simulink model "asw_28_simulator"  (R2018b)
settings: Solver=ode4  StartTime=0.0  StopTime=100  FixedStep=0.001  RelTol=1e-3
undefined symbols (not defined in the file): Earth, WGS84
libraries: simulink x4, aerolibutil x3, sharedtransform x2, aerolibtransform2 x2, aerolibfltsims x1, sharedutil x1
settings Model: Creator=benma  LastModifiedBy=benma

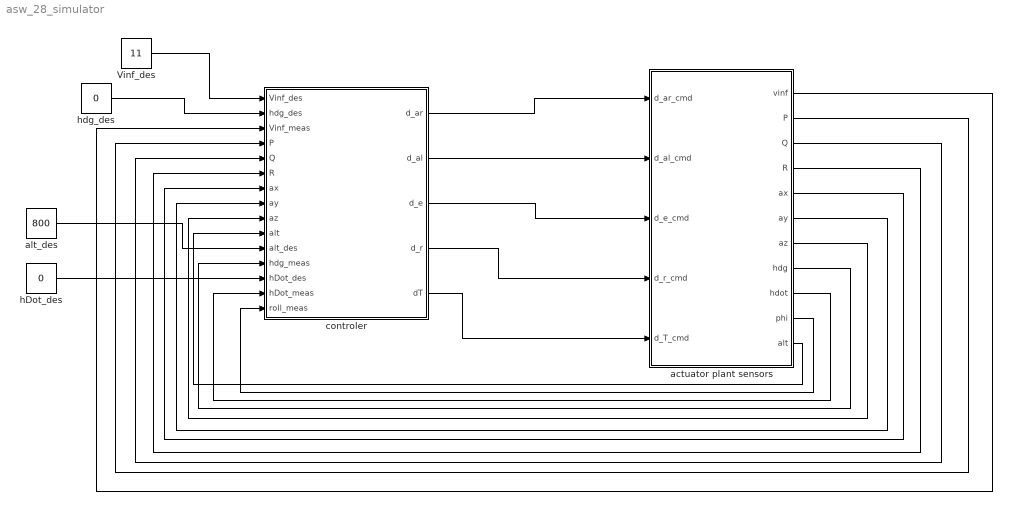
== system asw_28_simulator ==
  Vinf_des : Constant  Value=11
  actuator plant sensors : Subsystem
  alt_des : Constant  Value=800
  controler : Subsystem
  hDot_des : Constant  Value=0
  hdg_des : Constant  Value=0
  wires:
  controler/1(d_ar) -> actuator plant sensors/1(d_ar_cmd)
  controler/3(d_e) -> actuator plant sensors/3(d_e_cmd)
  controler/2(d_al) -> actuator plant sensors/2(d_al_cmd)
  controler/4(d_r) -> actuator plant sensors/4(d_r_cmd)
  hDot_des/1 -> controler/13(hDot_des)
  actuator plant sensors/9(hdot) -> controler/14(hDot_meas)
  actuator plant sensors/5(ax) -> controler/7(ax)
  actuator plant sensors/10(phi) -> controler/15(roll_meas)
  actuator plant sensors/3(Q) -> controler/5(Q)
  actuator plant sensors/4(R) -> controler/6(R)
  actuator plant sensors/2(P) -> controler/4(P)
  actuator plant sensors/6(ay) -> controler/8(ay)
  actuator plant sensors/1(vinf) -> controler/3(Vinf_meas)
  actuator plant sensors/7(az) -> controler/9(az)
  actuator plant sensors/8(hdg) -> controler/12(hdg_meas)
  hdg_des/1 -> controler/2(hdg_des)
  Vinf_des/1 -> controler/1(Vinf_des)
  actuator plant sensors/11(alt) -> controler/10(alt)
  alt_des/1 -> controler/11(alt_des)
  controler/5(dT) -> actuator plant sensors/5(d_T_cmd)

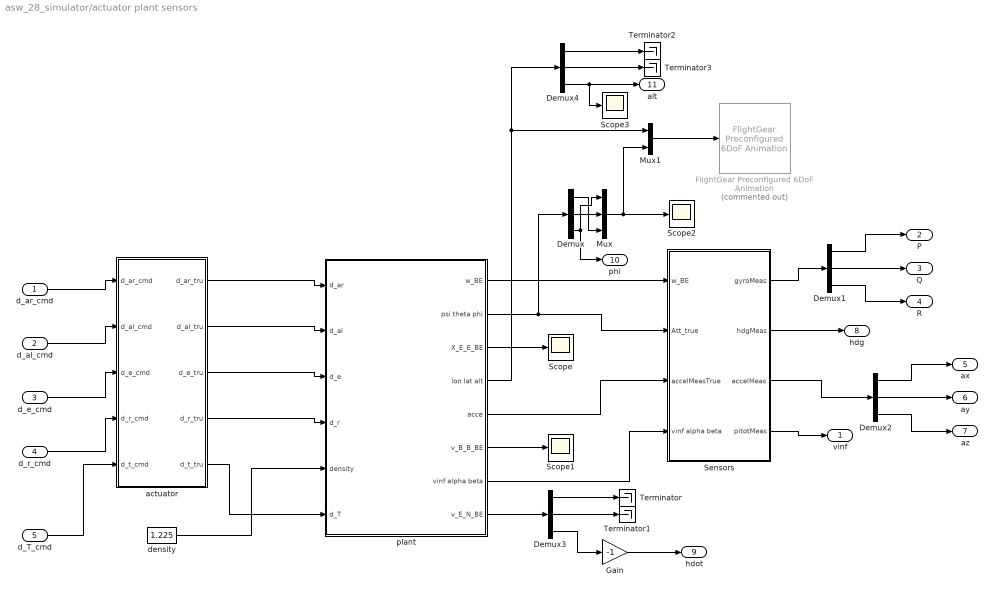
== system asw_28_simulator/actuator plant sensors ==
  d_ar_cmd : Inport
  d_al_cmd : Inport  Port=2
  d_e_cmd : Inport  Port=3
  d_r_cmd : Inport  Port=4
  d_T_cmd : Inport  Port=5
  Demux{,1..4} (5 alike) : Demux  Outputs=3
  FlightGear Preconfigured 6DoF Animation : aerolibfltsims/FlightGear Preconfigured 6DoF Animation  Commented=on  xFlightGearVersion=v2018.1  DestinationIpAddress=127.0.0.1  DestinationPort=5502  SampleTime=1/30  packetVersion=24
      settings: SourceProductName=Aerospace Blockset
  Gain : Gain  Gain=-1
  Mux : Mux  Inputs=3
  Mux1 : Mux  Inputs=2
  Scope{,1..3} (4 alike) : Scope
  Sensors : Subsystem
  Terminator{,1..3} (4 alike) : Terminator
  actuator : Subsystem
  density : Constant  Value=1.225
  plant : Subsystem
  vinf : Outport
  P : Outport  Port=2
  Q : Outport  Port=3
  R : Outport  Port=4
  ax : Outport  Port=5
  ay : Outport  Port=6
  az : Outport  Port=7
  hdg : Outport  Port=8
  hdot : Outport  Port=9
  phi : Outport  Port=10
  alt : Outport  Port=11
  wires:
  plant/6(v_B_B_BE) -> Scope1/1
  Demux/1 -> Mux/3
  Demux2/1 -> ax/1
  plant/4(lon lat alt) -> Mux1/1, Demux4/1
  plant/5(acce) -> Sensors/3(accelMeasTrue)
  d_e_cmd/1 -> actuator/3(d_e_cmd)
  Sensors/3(accelMeas) -> Demux2/1
  d_ar_cmd/1 -> actuator/1(d_ar_cmd)
  Sensors/2(hdgMeas) -> hdg/1
  Mux1/1 -> FlightGear Preconfigured 6DoF Animation/1
  actuator/3(d_e_tru) -> plant/3(d_e)
  plant/7(vinf alpha beta) -> Sensors/4(vinf alpha beta)
  Demux1/1 -> P/1
  d_r_cmd/1 -> actuator/4(d_r_cmd)
  actuator/1(d_ar_tru) -> plant/1(d_ar)
  plant/3(X_E_E_BE) -> Scope/1
  Demux1/3 -> R/1
  plant/1(w_BE) -> Sensors/1(w_BE)
  density/1 -> plant/5(density)
  Sensors/1(gyroMeas) -> Demux1/1
  Mux/1 -> Scope2/1, Mux1/2
  actuator/2(d_al_tru) -> plant/2(d_al)
  Demux/2 -> Mux/2
  Demux2/2 -> ay/1
  Demux1/2 -> Q/1
  plant/2(psi theta phi) -> Sensors/2(Att_true), Demux/1
  Sensors/4(pitotMeas) -> vinf/1
  Demux2/3 -> az/1
  d_al_cmd/1 -> actuator/2(d_al_cmd)
  actuator/4(d_r_tru) -> plant/4(d_r)
  Demux/3 -> phi/1, Mux/1
  plant/8(v_E_N_BE) -> Demux3/1
  Demux3/1 -> Terminator/1
  Demux3/2 -> Terminator1/1
  Demux3/3 -> Gain/1
  Gain/1 -> hdot/1
  Demux4/1 -> Terminator2/1
  Demux4/2 -> Terminator3/1
  Demux4/3 -> Scope3/1, alt/1
  d_T_cmd/1 -> actuator/5(d_t_cmd)
  actuator/5(d_t_tru) -> plant/6(d_T)

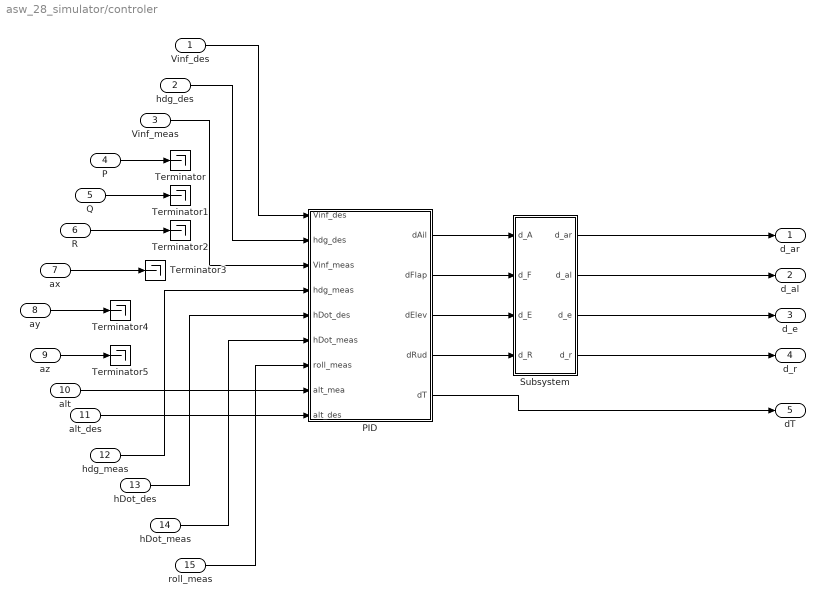
== system asw_28_simulator/controler ==
  Vinf_des : Inport
  hdg_des : Inport  Port=2
  Vinf_meas : Inport  Port=3
  P : Inport  Port=4
  Q : Inport  Port=5
  R : Inport  Port=6
  ax : Inport  Port=7
  ay : Inport  Port=8
  az : Inport  Port=9
  alt : Inport  Port=10
  alt_des : Inport  Port=11
  hdg_meas : Inport  Port=12
  hDot_des : Inport  Port=13
  hDot_meas : Inport  Port=14
  roll_meas : Inport  Port=15
  PID : Subsystem
  Subsystem : Subsystem
  Terminator{,1..5} (6 alike) : Terminator
  d_ar : Outport
  d_al : Outport  Port=2
  d_e : Outport  Port=3
  d_r : Outport  Port=4
  dT : Outport  Port=5
  wires:
  hdg_des/1 -> PID/2(hdg_des)
  Subsystem/2(d_al) -> d_al/1
  Vinf_des/1 -> PID/1(Vinf_des)
  Subsystem/3(d_e) -> d_e/1
  Vinf_meas/1 -> PID/3(Vinf_meas)
  hDot_des/1 -> PID/5(hDot_des)
  roll_meas/1 -> PID/7(roll_meas)
  Subsystem/4(d_r) -> d_r/1
  hdg_meas/1 -> PID/4(hdg_meas)
  PID/2(dFlap) -> Subsystem/2(d_F)
  Subsystem/1(d_ar) -> d_ar/1
  PID/4(dRud) -> Subsystem/4(d_R)
  PID/5(dT) -> dT/1
  PID/1(dAil) -> Subsystem/1(d_A)
  hDot_meas/1 -> PID/6(hDot_meas)
  PID/3(dElev) -> Subsystem/3(d_E)
  P/1 -> Terminator/1
  Q/1 -> Terminator1/1
  R/1 -> Terminator2/1
  ax/1 -> Terminator3/1
  ay/1 -> Terminator4/1
  az/1 -> Terminator5/1
  alt/1 -> PID/8(alt_mea)
  alt_des/1 -> PID/9(alt_des)

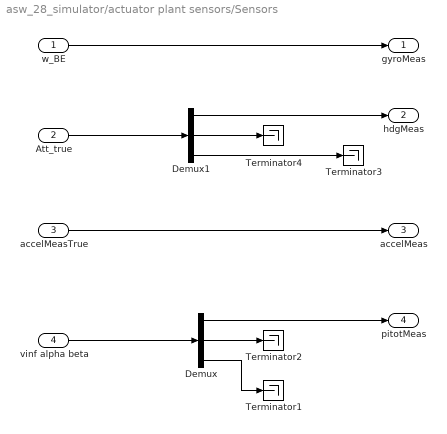
== system asw_28_simulator/actuator plant sensors/Sensors ==
  w_BE : Inport
  Att_true : Inport  Port=2
  accelMeasTrue : Inport  Port=3
  vinf alpha beta : Inport  Port=4
  Demux : Demux  Outputs=3
  Demux1 : Demux  Outputs=3
  Terminator{1..4} (4 alike) : Terminator
  gyroMeas : Outport
  hdgMeas : Outport  Port=2
  accelMeas : Outport  Port=3
  pitotMeas : Outport  Port=4
  wires:
  w_BE/1 -> gyroMeas/1
  vinf alpha beta/1 -> Demux/1
  Demux/3 -> Terminator1/1
  Demux/2 -> Terminator2/1
  Demux/1 -> pitotMeas/1
  accelMeasTrue/1 -> accelMeas/1
  Att_true/1 -> Demux1/1
  Demux1/2 -> Terminator4/1
  Demux1/1 -> hdgMeas/1
  Demux1/3 -> Terminator3/1

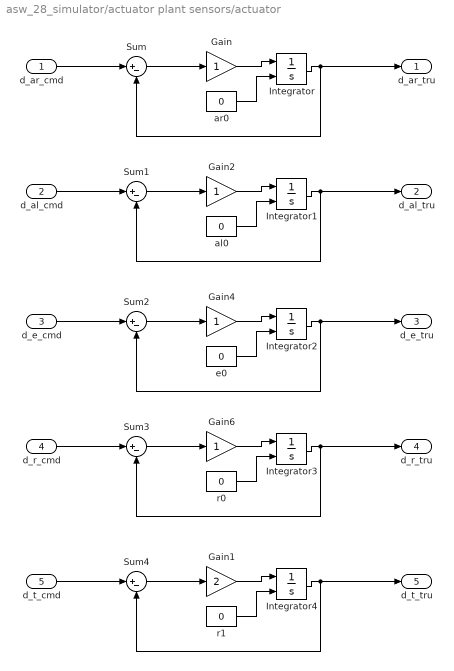
== system asw_28_simulator/actuator plant sensors/actuator ==
  d_ar_cmd : Inport
  d_al_cmd : Inport  Port=2
  d_e_cmd : Inport  Port=3
  d_r_cmd : Inport  Port=4
  d_t_cmd : Inport  Port=5
  Gain{,2,4,6} (4 alike) : Gain
  Gain1 : Gain  Gain=2
  Integrator{,1..4} (5 alike) : Integrator  InitialConditionSource=external
  Sum{,1..4} (5 alike) : Sum  Inputs=|+-
  al0 : Constant  Value=0
  ar0 : Constant  Value=0
  e0 : Constant  Value=0
  r0 : Constant  Value=0
  r1 : Constant  Value=0
  d_ar_tru : Outport
  d_al_tru : Outport  Port=2
  d_e_tru : Outport  Port=3
  d_r_tru : Outport  Port=4
  d_t_tru : Outport  Port=5
  wires:
  Sum/1 -> Gain/1
  d_ar_cmd/1 -> Sum/1
  Integrator/1 -> Sum/2, d_ar_tru/1
  Gain/1 -> Integrator/1
  d_al_cmd/1 -> Sum1/1
  Gain2/1 -> Integrator1/1
  Sum1/1 -> Gain2/1
  Integrator1/1 -> Sum1/2, d_al_tru/1
  d_e_cmd/1 -> Sum2/1
  Gain4/1 -> Integrator2/1
  Sum2/1 -> Gain4/1
  Integrator2/1 -> Sum2/2, d_e_tru/1
  d_r_cmd/1 -> Sum3/1
  Gain6/1 -> Integrator3/1
  Sum3/1 -> Gain6/1
  Integrator3/1 -> Sum3/2, d_r_tru/1
  ar0/1 -> Integrator/2
  al0/1 -> Integrator1/2
  e0/1 -> Integrator2/2
  r0/1 -> Integrator3/2
  d_t_cmd/1 -> Sum4/1
  Gain1/1 -> Integrator4/1
  r1/1 -> Integrator4/2
  Integrator4/1 -> Sum4/2, d_t_tru/1
  Sum4/1 -> Gain1/1

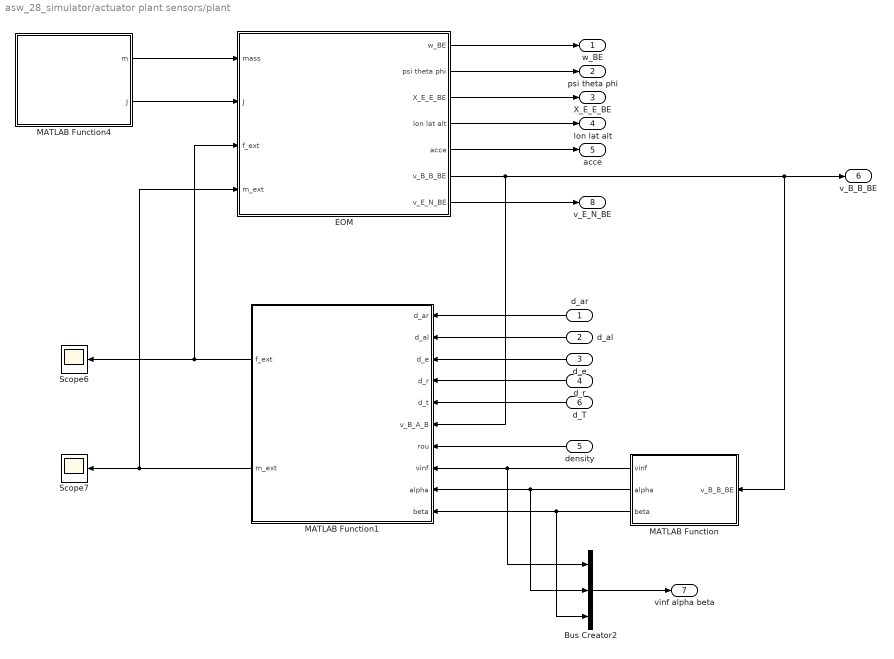
== system asw_28_simulator/actuator plant sensors/plant ==
  d_ar : Inport
  d_al : Inport  Port=2
  d_e : Inport  Port=3
  d_r : Inport  Port=4
  density : Inport  Port=5
  d_T : Inport  Port=6
  Bus Creator2 : BusCreator  Inputs=3
  EOM : Subsystem
  MATLAB Function : MATLAB Function  TreatAsAtomicUnit=on
  MATLAB Function1 : MATLAB Function  TreatAsAtomicUnit=on
  MATLAB Function4 : MATLAB Function  TreatAsAtomicUnit=on
  Scope6 : Scope
  Scope7 : Scope
  w_BE : Outport
  psi theta phi : Outport  Port=2
  X_E_E_BE : Outport  Port=3
  lon lat alt : Outport  Port=4
  acce : Outport  Port=5
  v_B_B_BE : Outport  Port=6
  vinf alpha beta : Outport  Port=7
  v_E_N_BE : Outport  Port=8
  wires:
  d_e/1 -> MATLAB Function1/3(d_e)
  d_al/1 -> MATLAB Function1/2(d_al)
  density/1 -> MATLAB Function1/7(rou)
  EOM/4(lon lat alt) -> lon lat alt/1
  EOM/2(psi theta phi) -> psi theta phi/1
  d_ar/1 -> MATLAB Function1/1(d_ar)
  MATLAB Function/3(beta) -> MATLAB Function1/10(beta), Bus Creator2/3
  EOM/1(w_BE) -> w_BE/1
  MATLAB Function/1(vinf) -> MATLAB Function1/8(vinf), Bus Creator2/1
  MATLAB Function1/1(f_ext) -> Scope6/1, EOM/3(f_ext)
  EOM/6(v_B_B_BE) -> MATLAB Function1/6(v_B_A_B), MATLAB Function/1(v_B_B_BE), v_B_B_BE/1
  EOM/3(X_E_E_BE) -> X_E_E_BE/1
  MATLAB Function/2(alpha) -> MATLAB Function1/9(alpha), Bus Creator2/2
  Bus Creator2/1 -> vinf alpha beta/1
  MATLAB Function4/1(m) -> EOM/1(mass)
  d_r/1 -> MATLAB Function1/4(d_r)
  MATLAB Function1/2(m_ext) -> Scope7/1, EOM/4(m_ext)
  MATLAB Function4/2(J) -> EOM/2(J)
  EOM/5(acce) -> acce/1
  EOM/7(v_E_N_BE) -> v_E_N_BE/1
  d_T/1 -> MATLAB Function1/5(d_t)

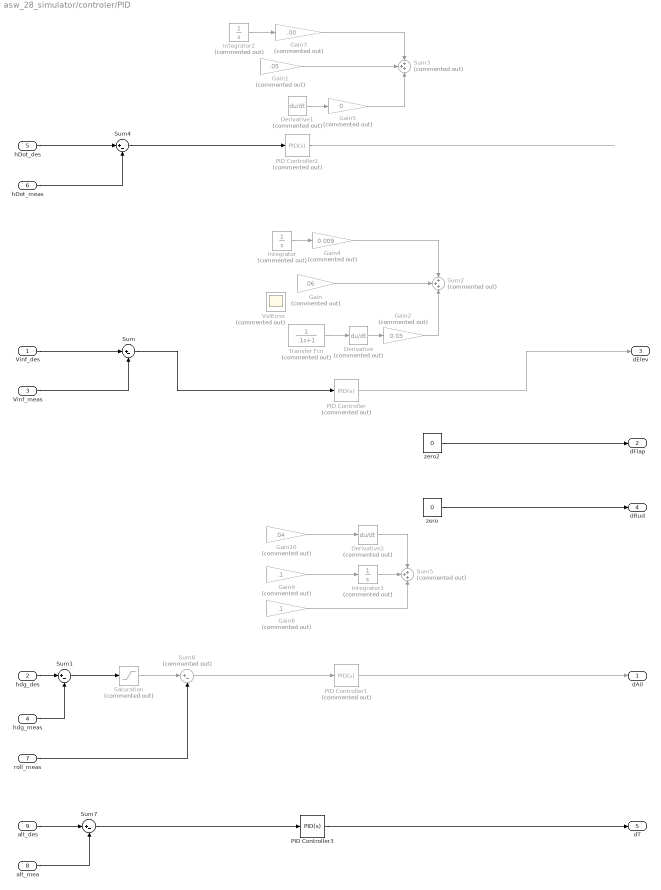
== system asw_28_simulator/controler/PID ==
  Vinf_des : Inport
  hdg_des : Inport  Port=2
  Vinf_meas : Inport  Port=3
  hdg_meas : Inport  Port=4
  hDot_des : Inport  Port=5
  hDot_meas : Inport  Port=6
  roll_meas : Inport  Port=7
  alt_mea : Inport  Port=8
  alt_des : Inport  Port=9
  Derivative : Derivative  Commented=on
  Derivative1 : Derivative  Commented=on
  Derivative2 : Derivative  Commented=on
  Gain : Gain  Commented=on  Gain=.06
  Gain1 : Gain  Commented=on  Gain=.05
  Gain10 : Gain  Commented=on  Gain=.04
  Gain2 : Gain  Commented=on  Gain=0.03
  Gain3 : Gain  Commented=on  Gain=.00
  Gain4 : Gain  Commented=on  Gain=0.009
  Gain5 : Gain  Commented=on  Gain=0
  Gain8 : Gain  Commented=on  Gain=.1
  Gain9 : Gain  Commented=on  Gain=.1
  Integrator : Integrator  Commented=on
  Integrator2 : Integrator  Commented=on
  Integrator3 : Integrator  Commented=on
  PID Controller : simulink/Continuous/PID Controller  Commented=on  Controller=PID  Form=Parallel  TimeDomain=Continuous-time  SampleTime=-1  IntegratorMethod=Forward Euler  FilterMethod=Forward Euler  ControllerParametersSource=internal  P=0  I=0.00458819667609101  D=0  UseFilter=on  N=100  TunerSelectOption=Transfer Function Based (PID Tuner App)  InitialConditionSource=internal  InitialConditionForIntegrator=0  InitialConditionForFilter=0  DifferentiatorICPrevScaledInput=0  ExternalReset=none  TrackingMode=off  Kt=1  LimitOutput=off  UpperSaturationLimit=inf  LowerSaturationLimit=-inf  LinearizeAsGain=on  AntiWindupMode=none  Kb=1  POutMin=[]  POutMax=[]  IOutMin=[]  IOutMax=[]  DOutMin=[]  DOutMax=[]  NOutMin=[]  NOutMax=[]  SumOutMin=[]  SumOutMax=[]  SaturationOutMin=[]  SaturationOutMax=[]  PParamMin=[]  PParamMax=[]  IParamMin=[]  IParamMax=[]  DParamMin=[]  DParamMax=[]  NParamMin=[]  NParamMax=[]  KbParamMin=[]  KbParamMax=[]  KtParamMin=[]  KtParamMax=[]  KbOutMin=[]  KbOutMax=[]  KtOutMin=[]  KtOutMax=[]  IntegratorOutMin=[]  IntegratorOutMax=[]  FilterOutMin=[]  FilterOutMax=[]  SumI1OutMin=[]  SumI1OutMax=[]  SumI2OutMin=[]  SumI2OutMax=[]  SumI3OutMin=[]  SumI3OutMax=[]  SumI4OutMin=[]  SumI4OutMax=[]  SumDOutMin=[]  SumDOutMax=[]  DifferentiatorOutMin=[]  DifferentiatorOutMax=[]  FilterDiffOutCoefMin=[]  FilterDiffOutCoefMax=[]  ReciprocalOutMin=[]  ReciprocalOutMax=[]  SumDenOutMin=[]  SumDenOutMax=[]  SumNumOutMin=[]  SumNumOutMax=[]  DivideOutMin=[]  DivideOutMax=[]  IntegratorContinuousStateAttributes=''  IntegratorStateMustResolveToSignalObject=off  IntegratorRTWStateStorageClass=Auto  FilterContinuousStateAttributes=''  FilterStateMustResolveToSignalObject=off  FilterRTWStateStorageClass=Auto  ParallelPVariant=InternalParameters  IdealPVariant=Disabled  IVariant=InternalParameters  DVariant=InternalParameters  IntegratorVariant=Continuous  SatVariant=Disabled  AWVariant=Passthrough  PCopyVariant=Disabled  TRVariant=Disabled  FdbkBlocksVariant=Forward  IdealPFdbkVariant=Disabled  SatFdbkVariant=Disabled  DerivativeFilterVariant=ContFilter  NVariant=InternalParameters  NCopyVariant=Disabled  FilterICVariant=InternalICsFilter  IntegratorICVariant=InternalICs  ExternalResetVariant=Disabled  TRSumVariant=Passthrough  SumFdbkVariant=Disabled  SumVariant=Sum_PID
  PID Controller1 : simulink/Continuous/PID Controller  Commented=on  Controller=PID  Form=Parallel  TimeDomain=Continuous-time  SampleTime=-1  IntegratorMethod=Forward Euler  FilterMethod=Forward Euler  ControllerParametersSource=internal  P=9.77454718036459e-06  I=1.32410445992676e-08  D=0.00160321592226225  UseFilter=on  N=26.5366033524893  TunerSelectOption=Transfer Function Based (PID Tuner App)  InitialConditionSource=internal  InitialConditionForIntegrator=0  InitialConditionForFilter=0  DifferentiatorICPrevScaledInput=0  ExternalReset=none  TrackingMode=off  Kt=1  LimitOutput=off  UpperSaturationLimit=inf  LowerSaturationLimit=-inf  LinearizeAsGain=on  AntiWindupMode=none  Kb=1  POutMin=[]  POutMax=[]  IOutMin=[]  IOutMax=[]  DOutMin=[]  DOutMax=[]  NOutMin=[]  NOutMax=[]  SumOutMin=[]  SumOutMax=[]  SaturationOutMin=[]  SaturationOutMax=[]  PParamMin=[]  PParamMax=[]  IParamMin=[]  IParamMax=[]  DParamMin=[]  DParamMax=[]  NParamMin=[]  NParamMax=[]  KbParamMin=[]  KbParamMax=[]  KtParamMin=[]  KtParamMax=[]  KbOutMin=[]  KbOutMax=[]  KtOutMin=[]  KtOutMax=[]  IntegratorOutMin=[]  IntegratorOutMax=[]  FilterOutMin=[]  FilterOutMax=[]  SumI1OutMin=[]  SumI1OutMax=[]  SumI2OutMin=[]  SumI2OutMax=[]  SumI3OutMin=[]  SumI3OutMax=[]  SumI4OutMin=[]  SumI4OutMax=[]  SumDOutMin=[]  SumDOutMax=[]  DifferentiatorOutMin=[]  DifferentiatorOutMax=[]  FilterDiffOutCoefMin=[]  FilterDiffOutCoefMax=[]  ReciprocalOutMin=[]  ReciprocalOutMax=[]  SumDenOutMin=[]  SumDenOutMax=[]  SumNumOutMin=[]  SumNumOutMax=[]  DivideOutMin=[]  DivideOutMax=[]  IntegratorContinuousStateAttributes=''  IntegratorStateMustResolveToSignalObject=off  IntegratorRTWStateStorageClass=Auto  FilterContinuousStateAttributes=''  FilterStateMustResolveToSignalObject=off  FilterRTWStateStorageClass=Auto  ParallelPVariant=InternalParameters  IdealPVariant=Disabled  IVariant=InternalParameters  DVariant=InternalParameters  IntegratorVariant=Continuous  SatVariant=Disabled  AWVariant=Passthrough  PCopyVariant=Disabled  TRVariant=Disabled  FdbkBlocksVariant=Forward  IdealPFdbkVariant=Disabled  SatFdbkVariant=Disabled  DerivativeFilterVariant=ContFilter  NVariant=InternalParameters  NCopyVariant=Disabled  FilterICVariant=InternalICsFilter  IntegratorICVariant=InternalICs  ExternalResetVariant=Disabled  TRSumVariant=Passthrough  SumFdbkVariant=Disabled  SumVariant=Sum_PID
  PID Controller2 : simulink/Continuous/PID Controller  Commented=on  Controller=PID  Form=Parallel  TimeDomain=Continuous-time  SampleTime=-1  IntegratorMethod=Forward Euler  FilterMethod=Forward Euler  ControllerParametersSource=internal  P=1  I=1  D=0  UseFilter=on  N=100  TunerSelectOption=Transfer Function Based (PID Tuner App)  InitialConditionSource=internal  InitialConditionForIntegrator=0  InitialConditionForFilter=0  DifferentiatorICPrevScaledInput=0  ExternalReset=none  TrackingMode=off  Kt=1  LimitOutput=off  UpperSaturationLimit=inf  LowerSaturationLimit=-inf  LinearizeAsGain=on  AntiWindupMode=none  Kb=1  POutMin=[]  POutMax=[]  IOutMin=[]  IOutMax=[]  DOutMin=[]  DOutMax=[]  NOutMin=[]  NOutMax=[]  SumOutMin=[]  SumOutMax=[]  SaturationOutMin=[]  SaturationOutMax=[]  PParamMin=[]  PParamMax=[]  IParamMin=[]  IParamMax=[]  DParamMin=[]  DParamMax=[]  NParamMin=[]  NParamMax=[]  KbParamMin=[]  KbParamMax=[]  KtParamMin=[]  KtParamMax=[]  KbOutMin=[]  KbOutMax=[]  KtOutMin=[]  KtOutMax=[]  IntegratorOutMin=[]  IntegratorOutMax=[]  FilterOutMin=[]  FilterOutMax=[]  SumI1OutMin=[]  SumI1OutMax=[]  SumI2OutMin=[]  SumI2OutMax=[]  SumI3OutMin=[]  SumI3OutMax=[]  SumI4OutMin=[]  SumI4OutMax=[]  SumDOutMin=[]  SumDOutMax=[]  DifferentiatorOutMin=[]  DifferentiatorOutMax=[]  FilterDiffOutCoefMin=[]  FilterDiffOutCoefMax=[]  ReciprocalOutMin=[]  ReciprocalOutMax=[]  SumDenOutMin=[]  SumDenOutMax=[]  SumNumOutMin=[]  SumNumOutMax=[]  DivideOutMin=[]  DivideOutMax=[]  IntegratorContinuousStateAttributes=''  IntegratorStateMustResolveToSignalObject=off  IntegratorRTWStateStorageClass=Auto  FilterContinuousStateAttributes=''  FilterStateMustResolveToSignalObject=off  FilterRTWStateStorageClass=Auto  ParallelPVariant=InternalParameters  IdealPVariant=Disabled  IVariant=InternalParameters  DVariant=InternalParameters  IntegratorVariant=Continuous  SatVariant=Disabled  AWVariant=Passthrough  PCopyVariant=Disabled  TRVariant=Disabled  FdbkBlocksVariant=Forward  IdealPFdbkVariant=Disabled  SatFdbkVariant=Disabled  DerivativeFilterVariant=ContFilter  NVariant=InternalParameters  NCopyVariant=Disabled  FilterICVariant=InternalICsFilter  IntegratorICVariant=InternalICs  ExternalResetVariant=Disabled  TRSumVariant=Passthrough  SumFdbkVariant=Disabled  SumVariant=Sum_PID
  PID Controller3 : simulink/Continuous/PID Controller  Controller=PID  Form=Parallel  TimeDomain=Continuous-time  SampleTime=-1  IntegratorMethod=Forward Euler  FilterMethod=Forward Euler  ControllerParametersSource=internal  P=0.0353413437245368  I=0.000338962204159574  D=-0.0634572537880452  UseFilter=on  N=0.539417705552614  TunerSelectOption=Transfer Function Based (PID Tuner App)  InitialConditionSource=internal  InitialConditionForIntegrator=0  InitialConditionForFilter=0  DifferentiatorICPrevScaledInput=0  ExternalReset=none  TrackingMode=off  Kt=1  LimitOutput=off  UpperSaturationLimit=inf  LowerSaturationLimit=-inf  LinearizeAsGain=on  AntiWindupMode=none  Kb=1  POutMin=[]  POutMax=[]  IOutMin=[]  IOutMax=[]  DOutMin=[]  DOutMax=[]  NOutMin=[]  NOutMax=[]  SumOutMin=[]  SumOutMax=[]  SaturationOutMin=[]  SaturationOutMax=[]  PParamMin=[]  PParamMax=[]  IParamMin=[]  IParamMax=[]  DParamMin=[]  DParamMax=[]  NParamMin=[]  NParamMax=[]  KbParamMin=[]  KbParamMax=[]  KtParamMin=[]  KtParamMax=[]  KbOutMin=[]  KbOutMax=[]  KtOutMin=[]  KtOutMax=[]  IntegratorOutMin=[]  IntegratorOutMax=[]  FilterOutMin=[]  FilterOutMax=[]  SumI1OutMin=[]  SumI1OutMax=[]  SumI2OutMin=[]  SumI2OutMax=[]  SumI3OutMin=[]  SumI3OutMax=[]  SumI4OutMin=[]  SumI4OutMax=[]  SumDOutMin=[]  SumDOutMax=[]  DifferentiatorOutMin=[]  DifferentiatorOutMax=[]  FilterDiffOutCoefMin=[]  FilterDiffOutCoefMax=[]  ReciprocalOutMin=[]  ReciprocalOutMax=[]  SumDenOutMin=[]  SumDenOutMax=[]  SumNumOutMin=[]  SumNumOutMax=[]  DivideOutMin=[]  DivideOutMax=[]  IntegratorContinuousStateAttributes=''  IntegratorStateMustResolveToSignalObject=off  IntegratorRTWStateStorageClass=Auto  FilterContinuousStateAttributes=''  FilterStateMustResolveToSignalObject=off  FilterRTWStateStorageClass=Auto  ParallelPVariant=InternalParameters  IdealPVariant=Disabled  IVariant=InternalParameters  DVariant=InternalParameters  IntegratorVariant=Continuous  SatVariant=Disabled  AWVariant=Passthrough  PCopyVariant=Disabled  TRVariant=Disabled  FdbkBlocksVariant=Forward  IdealPFdbkVariant=Disabled  SatFdbkVariant=Disabled  DerivativeFilterVariant=ContFilter  NVariant=InternalParameters  NCopyVariant=Disabled  FilterICVariant=InternalICsFilter  IntegratorICVariant=InternalICs  ExternalResetVariant=Disabled  TRSumVariant=Passthrough  SumFdbkVariant=Disabled  SumVariant=Sum_PID
  Saturation : Saturate  Commented=on  UpperLimit=0.3  LowerLimit=-0.3
  Sum{,1,4,7} (4 alike) : Sum  Inputs=|+-
  Sum2 : Sum  Commented=on  Inputs=+++
  Sum3 : Sum  Commented=on  Inputs=+++
  Sum5 : Sum  Commented=on  Inputs=+++
  Sum6 : Sum  Commented=on  Inputs=|+-
  Transfer Fcn : TransferFcn  Commented=on  Denominator=[.1 1]
  VelError : Scope  Commented=on
  zero : Constant  Value=0
  zero2 : Constant  Value=0
  dAil : Outport
  dFlap : Outport  Port=2
  dElev : Outport  Port=3
  dRud : Outport  Port=4
  dT : Outport  Port=5
  wires:
  zero2/1 -> dFlap/1
  zero/1 -> dRud/1
  Gain/1 -> Sum2/2
  Vinf_des/1 -> Sum/1
  ? -> VelError/1, Transfer Fcn/1, Gain/1, Integrator/1
  hdg_des/1 -> Sum1/1
  Integrator/1 -> Gain4/1
  Gain4/1 -> Sum2/1
  Derivative/1 -> Gain2/1
  Gain2/1 -> Sum2/3
  Vinf_meas/1 -> Sum/2
  Transfer Fcn/1 -> Derivative/1
  hdg_meas/1 -> Sum1/2
  hDot_des/1 -> Sum4/1
  hDot_meas/1 -> Sum4/2
  ? -> Derivative1/1, Gain1/1, Integrator2/1
  Integrator2/1 -> Gain3/1
  Gain3/1 -> Sum3/1
  ? -> Gain8/1, Gain10/1, Gain9/1
  Gain8/1 -> Sum5/3
  Gain9/1 -> Integrator3/1
  Integrator3/1 -> Sum5/2
  PID Controller1/1 -> dAil/1
  Gain10/1 -> Derivative2/1
  Derivative2/1 -> Sum5/1
  roll_meas/1 -> Sum6/2
  PID Controller2/1 -> ?
  Gain1/1 -> Sum3/2
  Gain5/1 -> Sum3/3
  Derivative1/1 -> Gain5/1
  PID Controller/1 -> dElev/1
  Sum/1 -> PID Controller/1
  Sum6/1 -> PID Controller1/1
  Sum1/1 -> Saturation/1
  Saturation/1 -> Sum6/1
  Sum4/1 -> PID Controller2/1
  alt_des/1 -> Sum7/1
  alt_mea/1 -> Sum7/2
  Sum7/1 -> PID Controller3/1
  PID Controller3/1 -> dT/1

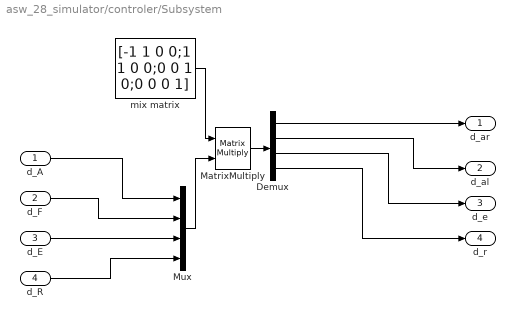
== system asw_28_simulator/controler/Subsystem ==
  d_A : Inport
  d_F : Inport  Port=2
  d_E : Inport  Port=3
  d_R : Inport  Port=4
  Demux : Demux
  MatrixMultiply : Product  Multiplication=Matrix(*)
  Mux : Mux
  mix matrix : Constant  Value=[-1 1 0 0;1 1 0 0;0 0 1 0;0 0 0 1]
  d_ar : Outport
  d_al : Outport  Port=2
  d_e : Outport  Port=3
  d_r : Outport  Port=4
  wires:
  d_E/1 -> Mux/3
  d_A/1 -> Mux/1
  Demux/3 -> d_e/1
  d_R/1 -> Mux/4
  d_F/1 -> Mux/2
  Demux/2 -> d_al/1
  MatrixMultiply/1 -> Demux/1
  Demux/4 -> d_r/1
  Demux/1 -> d_ar/1
  Mux/1 -> MatrixMultiply/2
  mix matrix/1 -> MatrixMultiply/1

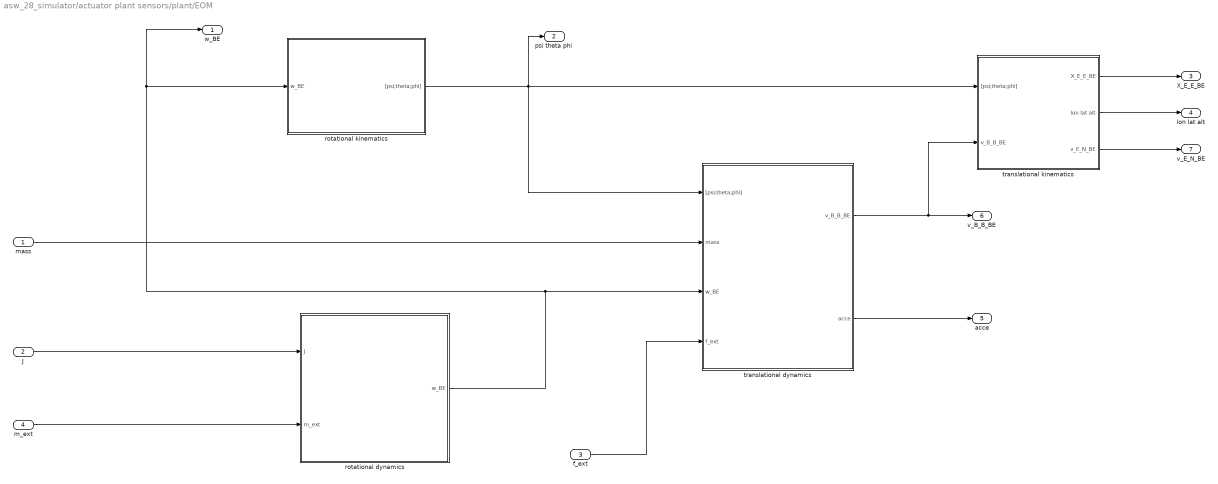
== system asw_28_simulator/actuator plant sensors/plant/EOM ==
  mass : Inport
  J : Inport  Port=2
  f_ext : Inport  Port=3
  m_ext : Inport  Port=4
  rotational dynamics : Subsystem
  rotational kinematics : Subsystem
  translational dynamics : Subsystem
  translational kinematics : Subsystem
  w_BE : Outport
  psi theta phi : Outport  Port=2
  X_E_E_BE : Outport  Port=3
  lon lat alt : Outport  Port=4
  acce : Outport  Port=5
  v_B_B_BE : Outport  Port=6
  v_E_N_BE : Outport  Port=7
  wires:
  J/1 -> rotational dynamics/1(J)
  mass/1 -> translational dynamics/2(mass)
  rotational dynamics/1(w_BE) -> translational dynamics/3(w_BE), w_BE/1, rotational kinematics/1(w_BE)
  translational kinematics/2(lon lat alt) -> lon lat alt/1
  f_ext/1 -> translational dynamics/4(f_ext)
  translational kinematics/1(X_E_E_BE) -> X_E_E_BE/1
  translational dynamics/1(v_B_B_BE) -> translational kinematics/2(v_B_B_BE), v_B_B_BE/1
  m_ext/1 -> rotational dynamics/2(m_ext)
  rotational kinematics/1("[psi;theta;phi]") -> psi theta phi/1, translational dynamics/1("[psi;theta;phi]"), translational kinematics/1("[psi;theta;phi]")
  translational dynamics/2(acce) -> acce/1
  translational kinematics/3(v_E_N_BE) -> v_E_N_BE/1

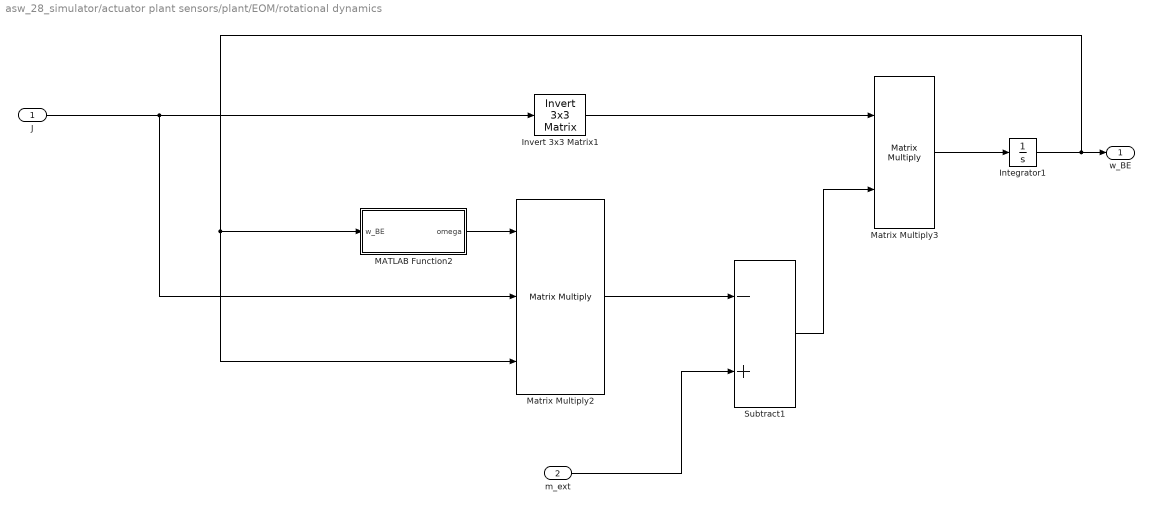
== system asw_28_simulator/actuator plant sensors/plant/EOM/rotational dynamics ==
  J : Inport
  m_ext : Inport  Port=2
  Integrator1 : Integrator  InitialCondition=[0;0;0]
  Invert 3x3 Matrix1 : aerolibutil/Invert  3x3 Matrix
  MATLAB Function2 : MATLAB Function  TreatAsAtomicUnit=on
  Matrix Multiply2 : Product  Inputs=3  Multiplication=Matrix(*)
  Matrix Multiply3 : Product  Multiplication=Matrix(*)
  Subtract1 : Sum  Inputs=-+
  w_BE : Outport
  wires:
  MATLAB Function2/1(omega) -> Matrix Multiply2/1
  J/1 -> Matrix Multiply2/2, Invert 3x3 Matrix1/1
  Matrix Multiply3/1 -> Integrator1/1
  Matrix Multiply2/1 -> Subtract1/1
  Subtract1/1 -> Matrix Multiply3/2
  m_ext/1 -> Subtract1/2
  Invert 3x3 Matrix1/1 -> Matrix Multiply3/1
  Integrator1/1 -> Matrix Multiply2/3, MATLAB Function2/1(w_BE), w_BE/1

== system asw_28_simulator/actuator plant sensors/plant/EOM/rotational kinematics ==
  w_BE : Inport
  Demux : Demux  Outputs=3
  Integrator2 : Integrator  InitialCondition=[0;0;0]
  MATLAB Function : MATLAB Function  TreatAsAtomicUnit=on
  MATLAB Function1 : MATLAB Function  TreatAsAtomicUnit=on
  Matrix Multiply4 : Product  Multiplication=Matrix(*)
  Mux : Mux  Inputs=3
  "[psi;theta;phi]" : Outport
  wires:
  MATLAB Function/1(tran) -> Matrix Multiply4/1
  MATLAB Function1/1(att) -> Demux/1, MATLAB Function/1(att)
  Matrix Multiply4/1 -> Integrator2/1
  w_BE/1 -> Matrix Multiply4/2
  Demux/2 -> Mux/2
  Mux/1 -> "[psi;theta;phi]"/1
  Demux/1 -> Mux/3
  Demux/3 -> Mux/1
  Integrator2/1 -> MATLAB Function1/1("att ")

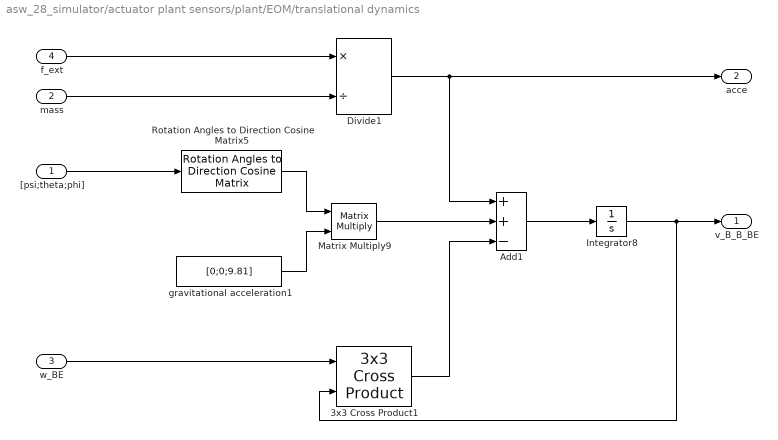
== system asw_28_simulator/actuator plant sensors/plant/EOM/translational dynamics ==
  "[psi;theta;phi]" : Inport
  mass : Inport  Port=2
  w_BE : Inport  Port=3
  f_ext : Inport  Port=4
  3x3 Cross Product1 : sharedutil/3x3 Cross Product  aMode=aMode
      settings: SourceProductBaseCode=AE
  Add1 : Sum  Inputs=++-
  Divide1 : Product  Inputs=*/
  Integrator8 : Integrator  InitialCondition=[13;0;0]
  Matrix Multiply9 : Product  Multiplication=Matrix(*)
  Rotation Angles to Direction Cosine Matrix5 : sharedtransform/Rotation Angles to Direction Cosine Matrix  rotationOrder=ZYX  aMode=aMode
      settings: SourceProductBaseCode=AE
  gravitational acceleration1 : Constant  Value=[0;0;9.81]
  v_B_B_BE : Outport
  acce : Outport  Port=2
  wires:
  "[psi;theta;phi]"/1 -> Rotation Angles to Direction Cosine Matrix5/1
  Matrix Multiply9/1 -> Add1/2
  mass/1 -> Divide1/2
  w_BE/1 -> 3x3 Cross Product1/1
  Divide1/1 -> acce/1, Add1/1
  gravitational acceleration1/1 -> Matrix Multiply9/2
  Add1/1 -> Integrator8/1
  Integrator8/1 -> 3x3 Cross Product1/2, v_B_B_BE/1
  f_ext/1 -> Divide1/1
  Rotation Angles to Direction Cosine Matrix5/1 -> Matrix Multiply9/1
  3x3 Cross Product1/1 -> Add1/3

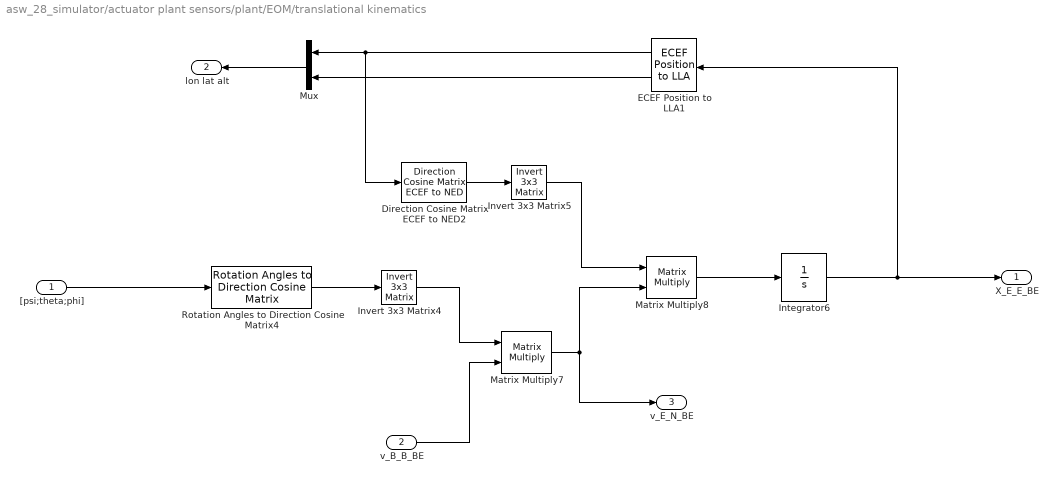
== system asw_28_simulator/actuator plant sensors/plant/EOM/translational kinematics ==
  "[psi;theta;phi]" : Inport
  v_B_B_BE : Inport  Port=2
  Direction Cosine Matrix ECEF to NED2 : aerolibtransform2/Direction Cosine Matrix ECEF to NED
      settings: SourceProductName=Aerospace Blockset  SourceProductBaseCode=AE
  ECEF Position to LLA1 : aerolibtransform2/ECEF Position to LLA  units=Metric (MKS)  ptype=Earth (WGS84)  F=1/298.257223563  R=6378137
      settings: SourceProductName=Aerospace Blockset  SourceProductBaseCode=AE
  Integrator6 : Integrator  InitialCondition=[6379000,0,0]
  Invert 3x3 Matrix4 : aerolibutil/Invert  3x3 Matrix
  Invert 3x3 Matrix5 : aerolibutil/Invert  3x3 Matrix
  Matrix Multiply7 : Product  Multiplication=Matrix(*)
  Matrix Multiply8 : Product  Multiplication=Matrix(*)
  Mux : Mux  Inputs=2
  Rotation Angles to Direction Cosine Matrix4 : sharedtransform/Rotation Angles to Direction Cosine Matrix  rotationOrder=ZYX  aMode=aMode
      settings: SourceProductBaseCode=AE
  X_E_E_BE : Outport
  lon lat alt : Outport  Port=2
  v_E_N_BE : Outport  Port=3
  wires:
  "[psi;theta;phi]"/1 -> Rotation Angles to Direction Cosine Matrix4/1
  Direction Cosine Matrix ECEF to NED2/1 -> Invert 3x3 Matrix5/1
  Integrator6/1 -> X_E_E_BE/1, ECEF Position to LLA1/1
  ECEF Position to LLA1/2 -> Mux/2
  ECEF Position to LLA1/1 -> Direction Cosine Matrix ECEF to NED2/1, Mux/1
  Invert 3x3 Matrix5/1 -> Matrix Multiply8/1
  Matrix Multiply7/1 -> Matrix Multiply8/2, v_E_N_BE/1
  v_B_B_BE/1 -> Matrix Multiply7/2
  Rotation Angles to Direction Cosine Matrix4/1 -> Invert 3x3 Matrix4/1
  Matrix Multiply8/1 -> Integrator6/1
  Invert 3x3 Matrix4/1 -> Matrix Multiply7/1
  Mux/1 -> lon lat alt/1

== matlab function asw_28_simulator/actuator plant sensors/plant/MATLAB Function ==
  data: v_B_B_BE input; vinf output; alpha output; beta output
function [vinf,alpha,beta] = body2wind(v_B_B_BE)
vinf = norm(v_B_B_BE);
alpha = atan2(v_B_B_BE(3),v_B_B_BE(1));
beta = asin(v_B_B_BE(2)/vinf);
end

== matlab function asw_28_simulator/actuator plant sensors/plant/EOM/rotational dynamics/MATLAB Function2 ==
  data: omega output; w_BE input
function omega = omega_BE(w_BE)
% w = (p;q;r)
omega = [0 -w_BE(3) w_BE(2);w_BE(3) 0 -w_BE(1);-w_BE(2) w_BE(1) 0];
end

== matlab function asw_28_simulator/actuator plant sensors/plant/MATLAB Function1 ==
  data: d_ar input; d_al input; d_e input; d_r input; d_t input; v_B_A_B input; rou input; f_ext output; m_ext output; vinf input; alpha input; beta input
function [f_ext,m_ext] = aeroSurface(d_ar,d_al,d_e,d_r,d_t,v_B_A_B,rou,vinf,alpha,beta)
%% Define Aircraft Mass and Geometry Properties (using grams)
%  mass       xSize     ySize     zSize    xLoc      yLoc       zLoc 
%  1          2         3         4        5         6          7
mng = ... %component of masses and geometry
  [90.0000    0.1000    0.9600    0.0100   -0.2300    0.4400         0;     %RightWing+Servo
   90.0000    0.1000    0.9600    0.0100   -0.2300   -0.4400         0;     %LeftWing+Servo
   13.0000    0.0750    0.3500    0.0020   -0.7600         0   -0.1600;     %Elevator
   72.0000    0.0650    0.0350    0.0150   -0.0500         0    0.0300;     %Battery
  106.0000    0.8700    0.0700    0.0700   -0.4000         0         0;     %Fuselage
   27.0000    0.0500    0.0300    0.0050   -0.0500         0    0.0200;     %Motor Controller
   10.0000    0.0400    0.0200    0.0050    0.1000         0    0.0200;     %Radio
   20.0000    0.0500    0.0100    0.0100   -0.0140         0         0;     %2 Servos
   40.0000    0.0300    0.0200    0.0200    0.0200         0    0.0100;     %Motor
   12.0000         0    0.2600    0.0250    0.0500         0    0.0100];    %Propeller
%%
% define total mass
m = sum(mng(:,1));
% define CG location
x_B_B_cmR = zeros(3,1);
x_B_B_cmR(1) = sum(mng(:,1).*mng(:,5))/sum(mng(:,1));
x_B_B_cmR(2) = sum(mng(:,1).*mng(:,6))/sum(mng(:,1));
x_B_B_cmR(3) = sum(mng(:,1).*mng(:,7))/sum(mng(:,1));
% define rotational inertia matrix
J = zeros(3,3);
cm_x = x_B_B_cmR(1)*ones(10,1);
cm_y = x_B_B_cmR(2)*ones(10,1);
cm_z = x_B_B_cmR(3)*ones(10,1);
J(1,1) = sum((mng(:,3).^2+mng(:,4).^2).*mng(:,1)/12+mng(:,1).*((mng(:,6)-cm_y).^2+(mng(:,7)-cm_z).^2));
J(2,2) = sum((mng(:,2).^2+mng(:,4).^2).*mng(:,1)/12+mng(:,1).*((mng(:,5)-cm_x).^2+(mng(:,7)-cm_z).^2));
J(3,3) = sum((mng(:,2).^2+mng(:,3).^2).*mng(:,1)/12+mng(:,1).*((mng(:,5)-cm_x).^2+(mng(:,6)-cm_y).^2));
J(1,2) = -sum(mng(:,1).*(mng(:,5)-cm_x).*(mng(:,6)-cm_y));
J(2,1) = J(1,2);
J(1,3) = -sum(mng(:,1).*(mng(:,5)-cm_x).*(mng(:,7)-cm_z));
J(3,1) = J(1,3);
J(2,3) = -sum(mng(:,1).*(mng(:,6)-cm_y).*(mng(:,7)-cm_z));
J(3,2) = J(2,3);
%% aero properties of surfaces
x_s2 = [-0.76,0,-0.16];%elevator
n_s2 = [0, 0, -1];
c_s2 = 0.075;
b_s2 = 0.35;
CL0_s2 = 0;
e_s2 = 0.8;
i_s2 = 0;
CD0_s2 = 0.01;
CDa_s2 = 1;
a0_s2 = 0;
CM0_s2 = 0;
CMa_s2 = 0;

x_s3 = [-0.76,0,-0.09];%rudder
n_s3 = [0, 1, 0];
c_s3 = 0.08;
b_s3 = 0.08;
CL0_s3 = 0;
e_s3 = 0.8;
i_s3 = 0;
CD0_s3 = 0.01;
CDa_s3 = 1;
a0_s3 = 0;
CM0_s3 = 0;
CMa_s3 = 0;

x_s4 = [-0.23,0.44,0];%right wing
n_s4 = [0, 0, -1];
c_s4 = 0.1;
b_s4 = 0.96;
CL0_s4 = 0.05;
e_s4 = 0.9;
i_s4 = 0.05;
CD0_s4 = 0.01;
CDa_s4 = 1;
a0_s4 = 0.05;
CM0_s4 = -0.05;
CMa_s4 = 0;

x_s5 = [-0.23,-0.44,0];%left wing
n_s5 = [0, 0, -1]; 
c_s5 = 0.1;
b_s5 = 0.96;
CL0_s5 = 0.05;
e_s5 = 0.9;
i_s5 = 0.05;
CD0_s5 = 0.01; 
CDa_s5 = 1;
a0_s5 = 0.05;
CM0_s5 = -0.05; 
CMa_s5 = 0;
%% convert data into matrix
x = [x_s2;x_s3;x_s4;x_s5];%position vector
n = [n_s2;n_s3;n_s4;n_s5];%normal vector
c = [c_s2;c_s3;c_s4;c_s5];%chord
b = [b_s2;b_s3;b_s4;b_s5];%span
CL0 = [CL0_s2;CL0_s3;CL0_s4;CL0_s5];%lift coef at aoa=0
e = [e_s2;e_s3;e_s4;e_s5];%osward efficiency factor
i = [i_s2;i_s3;i_s4;i_s5];%incidence aoa
d_u = [d_e;d_r;d_ar;d_al];%control surface deflection
CD0 = [CD0_s2;CD0_s3;CD0_s4;CD0_s5];%drag coef at aoa=0
CDa = [CDa_s2;CDa_s3;CDa_s4;CDa_s5];%drag coef deri w.r.t aoa
a0 = [a0_s2;a0_s3;a0_s4;a0_s5];%minimum drag aoa
CM0 = [CM0_s2;CM0_s3;CM0_s4;CM0_s5];%moment coef at aoa=0
CMa = [CMa_s2;CMa_s3;CMa_s4;CMa_s5];%moment coef deri w.r.t aoa
%%
%calculate parameters
aoa = i - asin(n*v_B_A_B/norm(v_B_A_B));%angle of attack of each surface
AR = b./c;%aspect ratio
S = b.*c;%area
CLa = 2*pi*AR./(2*ones(4,1)+AR);
CL = CL0+CLa.*aoa+3*d_u*0.1;
CD = CD0+CDa.*(aoa-a0).^2+CL.^2/pi./e./AR;
CM = CM0+CMa.*aoa;
%calculate for forces and moments on each surface
DyP = 0.5*rou*vinf^2;
L = CL*DyP.*S;
D = CD*DyP.*S;
M = CM.*DyP.*S.*c;
D_fu = 0.75*DyP*0.001;
F_s = zeros(3,4);
F_tot = [d_t-D_fu;0;0];
M_tot = [0;0;0];
C_W_B = [cos(beta) sin(beta) 0;-sin(beta) cos(beta) 0;0 0 1]*[cos(alpha) 0 sin(alpha);0 1 0;-sin(alpha) 0 cos(alpha)];
C_B_W = C_W_B';
for i = 1:4
    qc = 0.25*c(i);
    F_s(:,i) = L(i)*(n(i,:))'-[D(i);0;0];
    F_sb = C_B_W*F_s(:,i);
    F_tot = F_sb+F_tot;
    M_sw = M(i)*[0,0,0;0,0,-1;0, 1,0]*(n(i,:))'+cross((x(i,:))'-x_B_B_cmR+[qc;0;0],F_sb);
    M_tot = M_sw+M_tot;
end

f_ext = F_tot;
m_ext = M_tot;

end

== matlab function asw_28_simulator/actuator plant sensors/plant/EOM/rotational kinematics/MATLAB Function ==
  data: tran output; att input
function tran = att2tran(att)
% att = [phi;theta;psi]
phi = att(1);
theta = att(2);
tran = [1 tan(theta)*sin(phi) tan(theta)*cos(phi);0 cos(phi) -sin(phi);0 sin(phi)/cos(theta) cos(phi)/cos(theta)];
end

== matlab function asw_28_simulator/actuator plant sensors/plant/MATLAB Function4 ==
  data: m output; J output
function [m,J] = asw28MassnGeometry()
%% Define Aircraft Mass and Geometry Properties (using grams)
%  mass       xSize     ySize     zSize    xLoc      yLoc       zLoc 
%  1          2         3         4        5         6          7
mng = ... %component of masses and geometry
  [90.0000    0.1000    0.9600    0.0100   -0.2300    0.4400         0;     %RightWing+Servo
   90.0000    0.1000    0.9600    0.0100   -0.2300   -0.4400         0;     %LeftWing+Servo
   13.0000    0.0750    0.3500    0.0020   -0.7600         0   -0.1600;     %Elevator
   72.0000    0.0650    0.0350    0.0150   -0.0500         0    0.0300;     %Battery
  106.0000    0.8700    0.0700    0.0700   -0.4000         0         0;     %Fuselage
   27.0000    0.0500    0.0300    0.0050   -0.0500         0    0.0200;     %Motor Controller
   10.0000    0.0400    0.0200    0.0050    0.1000         0    0.0200;     %Radio
   20.0000    0.0500    0.0100    0.0100   -0.0140         0         0;     %2 Servos
   40.0000    0.0300    0.0200    0.0200    0.0200         0    0.0100;     %Motor
   12.0000         0    0.2600    0.0250    0.0500         0    0.0100];    %Propeller
%%
% define total mass
m = sum(mng(:,1))/1000;
% define CG location
x_B_B_cmR = zeros(3,1);
x_B_B_cmR(1) = sum(mng(:,1).*mng(:,5))/sum(mng(:,1));
x_B_B_cmR(2) = sum(mng(:,1).*mng(:,6))/sum(mng(:,1));
x_B_B_cmR(3) = sum(mng(:,1).*mng(:,7))/sum(mng(:,1));
% define rotational inertia matrix
J = zeros(3,3);
cm_x = x_B_B_cmR(1)*ones(10,1);
cm_y = x_B_B_cmR(2)*ones(10,1);
cm_z = x_B_B_cmR(3)*ones(10,1);
J(1,1) = sum((mng(:,3).^2+mng(:,4).^2).*mng(:,1)/12+mng(:,1).*((mng(:,6)-cm_y).^2+(mng(:,7)-cm_z).^2));
J(2,2) = sum((mng(:,2).^2+mng(:,4).^2).*mng(:,1)/12+mng(:,1).*((mng(:,5)-cm_x).^2+(mng(:,7)-cm_z).^2));
J(3,3) = sum((mng(:,2).^2+mng(:,3).^2).*mng(:,1)/12+mng(:,1).*((mng(:,5)-cm_x).^2+(mng(:,6)-cm_y).^2));
J(1,2) = -sum(mng(:,1).*(mng(:,5)-cm_x).*(mng(:,6)-cm_y));
J(2,1) = J(1,2);
J(1,3) = -sum(mng(:,1).*(mng(:,5)-cm_x).*(mng(:,7)-cm_z));
J(3,1) = J(1,3);
J(2,3) = -sum(mng(:,1).*(mng(:,6)-cm_y).*(mng(:,7)-cm_z));
J(3,2) = J(2,3);
J = J/1000;
end

== matlab function asw_28_simulator/actuator plant sensors/plant/EOM/rotational kinematics/MATLAB Function1 ==
  data: att input; att output
function att = attbound(att)
if att(1) >= pi
    att(1) = att(1)-2*pi;
elseif att(1) <= -pi
    att(1) = 2*pi+att(1);
end
if att(2) >= pi
    att(2) = att(2)-2*pi;
elseif att(2) <= -pi
    att(2) = 2*pi+att(2);
end
if att(3) >= pi
    att(3) = att(3)-2*pi;
elseif att(3) <= -pi
    att(3) = 2*pi+att(3);
end
end
